simulink library "DYN_GRAV"  (Simulink 9.0)
settings: Solver=VariableStepAuto  StartTime=0.0  StopTime=10.0  RelTol=1e-3
undefined symbols (not defined in the file): CONSTANTS_par, DYN_SC_par
libraries: LIB_ROT x7, LIB_ENV x1
settings Model: Creator=WilTravis  LastModifiedBy=Mahal

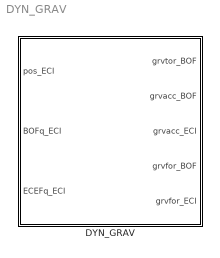
== system DYN_GRAV ==
  DYN_GRAV : Subsystem

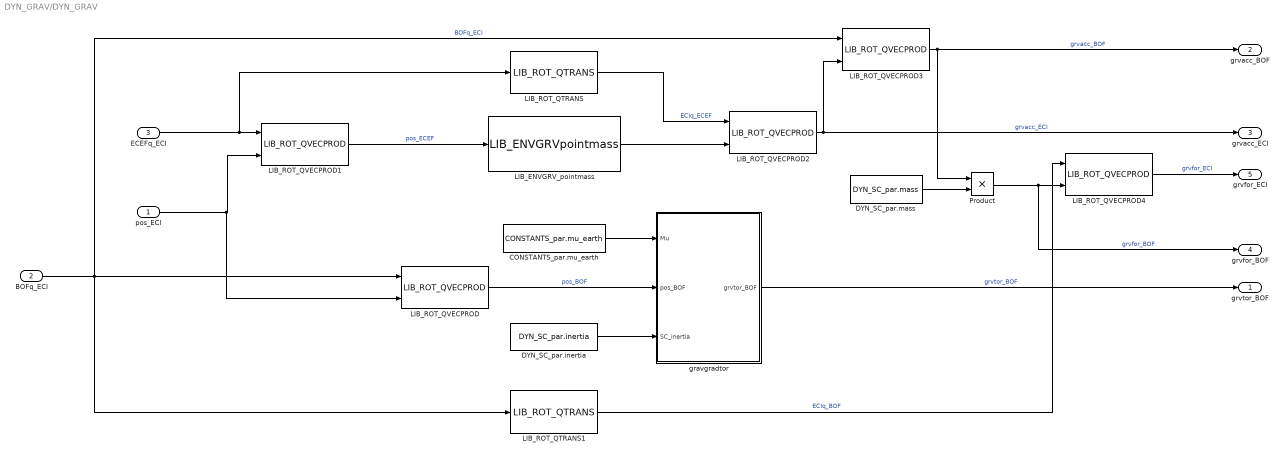
== system DYN_GRAV/DYN_GRAV ==
  pos_ECI : Inport
  BOFq_ECI : Inport  Port=2
  ECEFq_ECI : Inport  Port=3
  CONSTANTS_par.mu_earth : Constant  Value=CONSTANTS_par.mu_earth
  DYN_SC_par.inertia : Constant  Value=DYN_SC_par.inertia
  DYN_SC_par.mass : Constant  Value=DYN_SC_par.mass
  LIB_ENVGRV_pointmass : LIB_ENV/LIB_ENVGRVpointmass  mu_cst=CONSTANTS_par.mu_earth
  LIB_ROT_QTRANS : LIB_ROT/LIB_ROT_QTRANS
  LIB_ROT_QTRANS1 : LIB_ROT/LIB_ROT_QTRANS
  LIB_ROT_QVECPROD{,1..4} (5 alike) : LIB_ROT/LIB_ROT_QVECPROD
  Product : Product
  gravgradtor : MATLAB Function  TreatAsAtomicUnit=on
  grvtor_BOF : Outport
  grvacc_BOF : Outport  Port=2
  grvacc_ECI : Outport  Port=3
  grvfor_BOF : Outport  Port=4
  grvfor_ECI : Outport  Port=5
  wires:
  LIB_ROT_QVECPROD/1 -> gravgradtor/2(pos_BOF)  "pos_BOF"
  DYN_SC_par.inertia/1 -> gravgradtor/3(SC_inertia)
  LIB_ROT_QVECPROD2/1 -> grvacc_ECI/1, LIB_ROT_QVECPROD3/2  "grvacc_ECI"
  LIB_ROT_QVECPROD1/1 -> LIB_ENVGRV_pointmass/1  "pos_ECEF"
  CONSTANTS_par.mu_earth/1 -> gravgradtor/1(Mu)
  ECEFq_ECI/1 -> LIB_ROT_QVECPROD1/1, LIB_ROT_QTRANS/1
  pos_ECI/1 -> LIB_ROT_QVECPROD1/2, LIB_ROT_QVECPROD/2
  LIB_ROT_QTRANS/1 -> LIB_ROT_QVECPROD2/1  "ECIq_ECEF"
  gravgradtor/1(grvtor_BOF) -> grvtor_BOF/1  "grvtor_BOF"
  LIB_ROT_QVECPROD3/1 -> Product/1, grvacc_BOF/1  "grvacc_BOF"
  LIB_ENVGRV_pointmass/1 -> LIB_ROT_QVECPROD2/2
  DYN_SC_par.mass/1 -> Product/2
  BOFq_ECI/1 -> LIB_ROT_QTRANS1/1, LIB_ROT_QVECPROD/1, LIB_ROT_QVECPROD3/1  "BOFq_ECI"
  Product/1 -> grvfor_BOF/1, LIB_ROT_QVECPROD4/2  "grvfor_BOF"
  LIB_ROT_QTRANS1/1 -> LIB_ROT_QVECPROD4/1  "ECIq_BOF"
  LIB_ROT_QVECPROD4/1 -> grvfor_ECI/1  "grvfor_ECI"

== matlab function DYN_GRAV/gravgradtor ==
  data: Mu input double; grvtor_BOF output double; pos_BOF input double; SC_inertia input double
function grvtor_BOF = gravgradtor(Mu,pos_BOF,SC_inertia)

pos_BOF_mag = sqrt(pos_BOF(1)^2+pos_BOF(2)^2+pos_BOF(3)^2);

o_unit = pos_BOF./pos_BOF_mag;


grvtor_BOF = (3*(Mu/pos_BOF_mag^3)*VecCross(o_unit))*SC_inertia*o_unit;

end
